simulink model "controller"  (R2026a)
settings: Solver=ode4  StopTime=30  FixedStep=0.01
InitFcn:
  | load("trim_results.mat"); load("linearized_model.mat"); load("pitch_gains.mat");
values from neighbouring files (symbols this model uses):
  A_lon = [-0.0360303805261 -0.00465064609556 -9.13680289331e-19 0 0 4.61199857178 -3.19054098728 -30.4696428942 0 -64.9999999999 -5.12696743012e-11 0.972361458622 ... (25 elements, 5x5)]    [linearized_model.mat]    (also in liniarizeModel.m = T * A_lon_raw * T)
  B_lon = [-2.4057652358  2.39605925807; -0.265251038833  0.000456139691379; -43.8215088816  0; 0  0; 0  0]    [linearized_model.mat]    (also in liniarizeModel.m = T * B_lon_raw)
  C_lon = [1 0 0 0 0 0 1 0 0 0 0 0 ... (25 elements, 5x5)]    [linearized_model.mat]    (also in liniarizeModel.m = eye(5))
  D_lon = [0  0; 0  0; 0  0; 0  0; 0  0]    [linearized_model.mat]    (also in liniarizeModel.m = zeros(5,2))
  del_t_trim = 0.488713859757    [pitch_gains.mat]
  Kd = 0.02    [pitch_gains.mat]
  Ki = 0.2    [pitch_gains.mat]
  Kp = 1    [pitch_gains.mat]
  Kq = 0.45    [pitch_gains.mat]
libraries: slpidlib x1
settings Model: Creator=sahil  LastModifiedBy=sahil

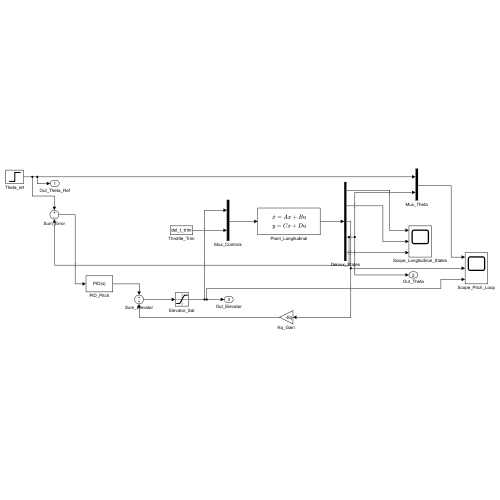
[thumbnail: Simulink's stored preview of the top-level diagram]
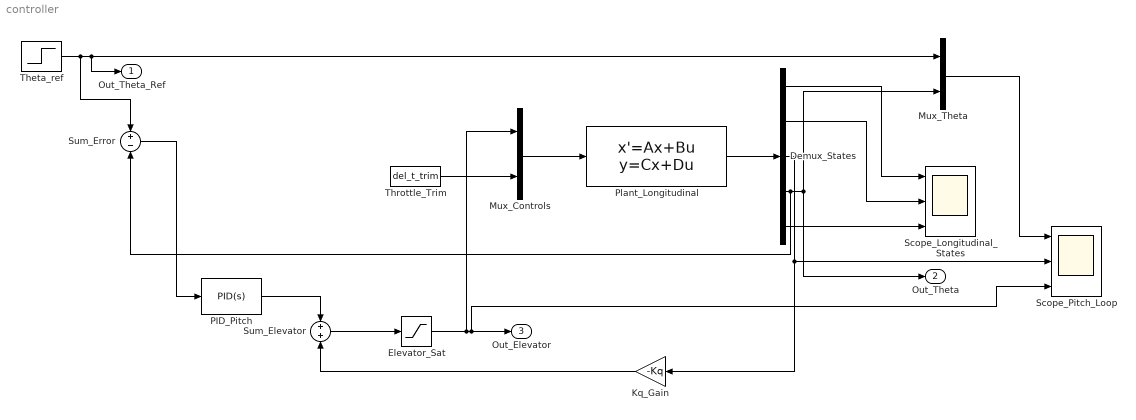
== system controller ==
  Demux_States : Demux  Outputs=5
  Elevator_Sat : Saturate  UpperLimit=25*pi/180  LowerLimit=-25*pi/180
  Kq_Gain : Gain  Gain=-Kq
  Mux_Controls : Mux  Inputs=2
  Mux_Theta : Mux  Inputs=2
  PID_Pitch : slpidlib/PID Controller  Controller=PID  Form=Parallel  TimeDomain=Continuous-time  UseExternalTs=off  SampleTime=-1  IntegratorMethod=Forward Euler  FilterMethod=Forward Euler  ControllerParametersSource=internal  P=Kp  I=Ki  UseKiTs=off  D=Kd  UseExternalDerivativeSource=off  N=100  UseFilter=on  TunerSelectOption=Transfer Function Based (PID Tuner App)  InitialConditionSource=internal  InitialConditionForIntegrator=0  InitialConditionForFilter=0  DifferentiatorICPrevScaledInput=0  ExternalReset=none  TrackingMode=off  Kt=1  LimitOutput=off  SatLimitsSource=internal  UpperSaturationLimit=inf  LowerSaturationLimit=-inf  LinearizeAsGain=on  AntiWindupMode=none  Kb=1  LimitIntegrator=off  UpperIntegratorSaturationLimit=inf  LowerIntegratorSaturationLimit=-inf  POutMin=[]  POutMax=[]  IOutMin=[]  IOutMax=[]  DOutMin=[]  DOutMax=[]  NOutMin=[]  NOutMax=[]  SumOutMin=[]  SumOutMax=[]  SaturationOutMin=[]  SaturationOutMax=[]  PParamMin=[]  PParamMax=[]  IParamMin=[]  IParamMax=[]  DParamMin=[]  DParamMax=[]  NParamMin=[]  NParamMax=[]  KbParamMin=[]  KbParamMax=[]  KtParamMin=[]  KtParamMax=[]  KbOutMin=[]  KbOutMax=[]  KtOutMin=[]  KtOutMax=[]  IntegratorOutMin=[]  IntegratorOutMax=[]  FilterOutMin=[]  FilterOutMax=[]  SumI1OutMin=[]  SumI1OutMax=[]  SumI2OutMin=[]  SumI2OutMax=[]  SumI3OutMin=[]  SumI3OutMax=[]  SumI4OutMin=[]  SumI4OutMax=[]  SumDOutMin=[]  SumDOutMax=[]  DifferentiatorOutMin=[]  DifferentiatorOutMax=[]  FilterDiffOutCoefMin=[]  FilterDiffOutCoefMax=[]  ReciprocalOutMin=[]  ReciprocalOutMax=[]  SumDenOutMin=[]  SumDenOutMax=[]  SumNumOutMin=[]  SumNumOutMax=[]  DivideOutMin=[]  DivideOutMax=[]  UdiffTsProdOutMin=[]  UdiffTsProdOutMax=[]  NTsProdOutMin=[]  NTsProdOutMax=[]  UintegralTsProdOutMin=[]  UintegralTsProdOutMax=[]  UngainTsProdOutMin=[]  UngainTsProdOutMax=[]  ClampingZeroOutDataTypeStr=Inherit: Inherit via back propagation  ClampingZeroOutMin=[]  ClampingZeroOutMax=[]  FilterDenConstantOutDataTypeStr=Inherit: Inherit via back propagation  FilterDenConstantOutMin=[]  FilterDenConstantOutMax=[]  PCopyOutDataTypeStr=Inherit: Inherit via back propagation  PCopyOutMin=[]  PCopyOutMax=[]  NCopyOutDataTypeStr=Inherit: Inherit via back propagation  NCopyOutMin=[]  NCopyOutMax=[]  IntegratorContinuousStateAttributes=''  IntegratorStateMustResolveToSignalObject=off  IntegratorRTWStateStorageClass=Auto  FilterContinuousStateAttributes=''  FilterStateMustResolveToSignalObject=off  FilterRTWStateStorageClass=Auto  ParallelPVariant=InternalParameters  IdealPVariant=Disabled  IVariant=InternalParameters  DVariant=InternalParameters  IntegratorVariant=Continuous  SatVariant=Disabled  AWVariant=Passthrough  PCopyVariant=Disabled  TRVariant=Disabled  FdbkBlocksVariant=Forward  IdealPFdbkVariant=Disabled  SatFdbkVariant=Disabled  DerivativeFilterVariant=ContFilter  NVariant=InternalParameters  NCopyVariant=Disabled  FilterICVariant=InternalICsFilter  IntegratorICVariant=InternalICs  ExternalResetVariant=Disabled  TRSumVariant=Passthrough  SumFdbkVariant=Disabled  SumVariant=Sum_PID  TsampFilterVariant=InternalTs  TsampNgainVariant=Passthrough  TsampIntegralVariant=Disabled_SignalSpec  ExternalSaturationOutDataTypeStr=Inherit: Same as second input  DerivativeSourceVariant=ErrorSignal  PreIntVariant=InternalPreInt
  Plant_Longitudinal : StateSpace  A=A_lon  B=B_lon  C=C_lon  D=D_lon  InitialCondition=0
  Scope_Longitudinal_States : Scope  NumInputPorts=3
  Scope_Pitch_Loop : Scope  NumInputPorts=3
      settings: ActiveDisplayYMinimum=-1.462731641683011  ActiveDisplayYMaximum=1.3096923899553046
  Sum_Elevator : Sum
  Sum_Error : Sum  Inputs=+-
  Theta_ref : Step  Time=5  FinalValue=5*pi/180  SampleTime=0
  Throttle_Trim : Constant  Value=del_t_trim
  Out_Theta_Ref : Outport
  Out_Theta : Outport  Port=2
  Out_Elevator : Outport  Port=3
  wires:
  Theta_ref/1 -> Mux_Theta/1, Out_Theta_Ref/1, Sum_Error/1
  Mux_Controls/1 -> Plant_Longitudinal/1
  Demux_States/2 -> Scope_Longitudinal_States/2
  Sum_Error/1 -> PID_Pitch/1
  Sum_Elevator/1 -> Elevator_Sat/1
  PID_Pitch/1 -> Sum_Elevator/1
  Throttle_Trim/1 -> Mux_Controls/2
  Kq_Gain/1 -> Sum_Elevator/2
  Elevator_Sat/1 -> Scope_Pitch_Loop/3, Out_Elevator/1, Mux_Controls/1
  Plant_Longitudinal/1 -> Demux_States/1
  Demux_States/1 -> Scope_Longitudinal_States/1
  Demux_States/3 -> Kq_Gain/1, Scope_Pitch_Loop/2
  Demux_States/4 -> Mux_Theta/2, Out_Theta/1, Sum_Error/2
  Demux_States/5 -> Scope_Longitudinal_States/3
  Mux_Theta/1 -> Scope_Pitch_Loop/1
